simulink model "dynamics"  (R2023b)
settings: Solver=ode45  StartTime=0.0  StopTime=StopTime  FixedStep=.1  RelTol=1e-5
PreLoadFcn:
  | StopTime = 5000; gravity = true; k = 10; b = 100; ktr = 300; btr = 300; d0 = 125; l0 = 515.3882; mu = 398600000000000; mp = 1500; mp_inv = 0.00066667; mtr = 1.6667; mtr_inv = 0.6; NRao0 = [-504.021290494982;4.21156034226775e-10;6878000]; NRbo0 = [504.021290495824;4.21156034226775e-10;6878000]; NRdo0 = [4.21156034226775e-10;-124.968757810126;6878000]; NReo0 = [4.21156034226775e-10;124.968757810969;6878000]; NVao0 = [-7612.67977015526;-3.08624030053628e-16;-5.04021290495356]; NVbo0 = [-7612.67977015526;3.08624030053685e-16;5.04021290495449]; NVdo0 = [-7612.67977015526;2.85429773939059e-29;4.66142195672722e-13]; NVeo0 = [-7612.67977015526;2.85429773939059e-29;4.66142195672722e-13];
undefined symbols (not defined in the file or in its folder): NRfo0, NRgo0, NVfo0, NVgo0
settings Model: Creator=cyrus  LastModifiedBy=cyrus

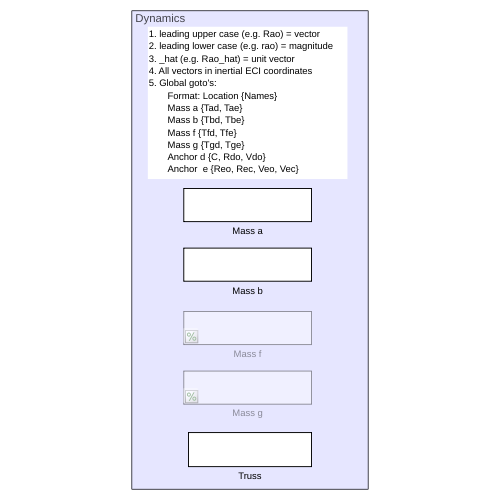
[thumbnail: Simulink's stored preview of the top-level diagram]
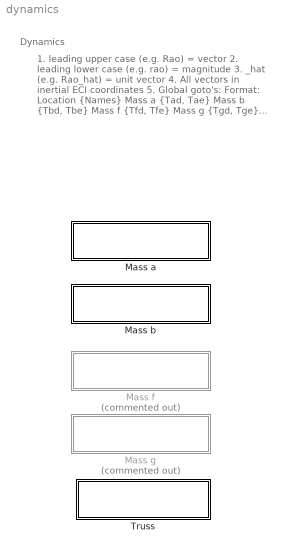
== system dynamics ==
  note: Dynamics
  note: 1. leading upper case (e.g. Rao) = vector
      | 2. leading lower case (e.g. rao) = magnitude
      | 3. _hat (e.g. Rao_hat) = unit vector
      | 4. All vectors in inertial ECI coordinates
      | 5. Global goto's:
      | 	Format: Location {Names}
      | 	Mass a {Tad, Tae}
      | 	Mass b {Tbd, Tbe}
      | 	Mass f {Tfd, Tfe}
      | 	Mass g {Tgd, Tge}
      | 	Anchor d {C, Rdo, Vdo}
      | 	Anchor  e {Reo, Rec, Veo, Vec}
  Mass a : Subsystem
  Mass b : Subsystem
  Mass f : Subsystem  Commented=on
  Mass g : Subsystem  Commented=on
  Truss : Subsystem

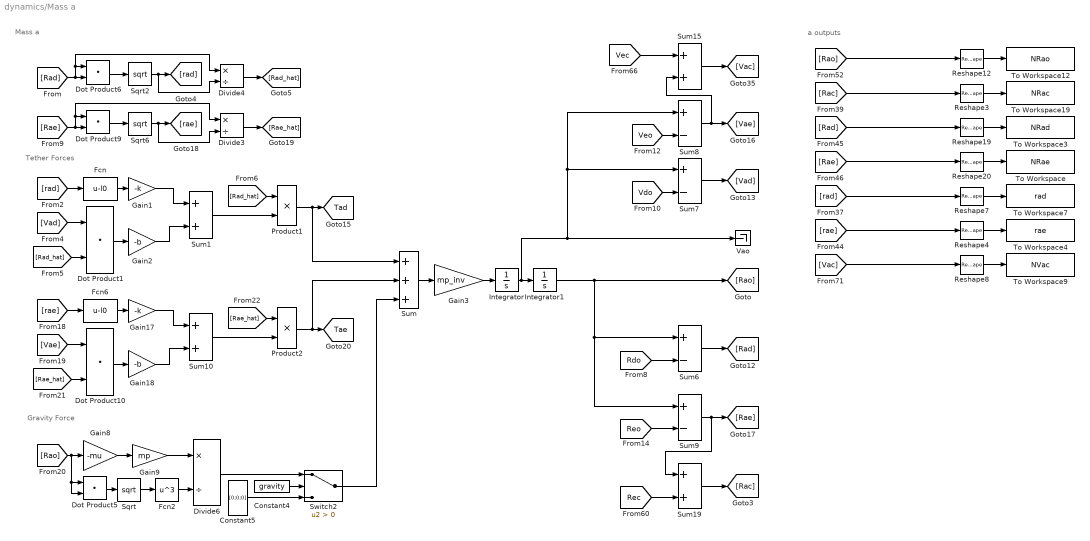
== system dynamics/Mass a ==
  note: Tether Forces
  note: Mass a
  note: Gravity Force
  note: a outputs
  Constant4 : Constant  Value=gravity
  Constant5 : Constant  Value=[0;0;0]  VectorParams1D=off
  Divide3 : Product  Inputs=*/
  Divide4 : Product  Inputs=*/
  Divide6 : Product  Inputs=*/
  Dot Product{1,5..6,9..10} (5 alike) : DotProduct  OutDataTypeStr=Inherit: Inherit via internal rule
  Fcn : Fcn  Expr=u-l0
  Fcn2 : Fcn  Expr=u^3
  Fcn6 : Fcn  Expr=u-l0
  Gain1 : Gain  Gain=-k
  Gain17 : Gain  Gain=-k
  Gain18 : Gain  Gain=-b
  Gain2 : Gain  Gain=-b
  Gain3 : Gain  Gain=mp_inv
  Gain8 : Gain  Gain=-mu
  Gain9 : Gain  Gain=mp
  Integrator : Integrator  InitialCondition=NVao0
  Integrator1 : Integrator  InitialCondition=NRao0
  Product1 : Product
  Product2 : Product
  Reshape{3..4,7..8,12,19..20} (7 alike) : Reshape
  Sqrt : Sqrt
  Sqrt2 : Sqrt
  Sqrt6 : Sqrt
  Sum : Sum  Inputs=+++
  Sum{1,10,15,19} (4 alike) : Sum
  Sum{6..9} (4 alike) : Sum  Inputs=+-
  Switch2 : Switch  Criteria=u2 > Threshold  SaturateOnIntegerOverflow=off  InputSameDT=off
  To Workspace : ToWorkspace  VariableName=NRae  SampleTime=-1
  To Workspace12 : ToWorkspace  VariableName=NRao  SampleTime=-1
      settings: Save2DSignal=2-D array (concatenate along first dimension)
  To Workspace19 : ToWorkspace  VariableName=NRac  SampleTime=-1
      settings: Save2DSignal=2-D array (concatenate along first dimension)
  To Workspace3 : ToWorkspace  VariableName=NRad  SampleTime=-1
  To Workspace4 : ToWorkspace  VariableName=rae  SampleTime=-1
      settings: Save2DSignal=2-D array (concatenate along first dimension)
  To Workspace7 : ToWorkspace  VariableName=rad  SampleTime=-1
      settings: Save2DSignal=2-D array (concatenate along first dimension)
  To Workspace9 : ToWorkspace  VariableName=NVac  SampleTime=-1
      settings: Save2DSignal=2-D array (concatenate along first dimension)
  Vao : Terminator
  tag scope: Tad=global, Tae=global
  wires:
  Sum19/1 -> [Rac]
  [rae] -> Fcn6/1
  [Rdo] -> Sum6/2
  Dot Product6/1 -> Sqrt2/1
  Gain17/1 -> Sum10/1
  [Veo] -> Sum8/2
  [Vec] -> Sum15/1
  Dot Product10/1 -> Gain18/1
  Dot Product5/1 -> Sqrt/1
  Gain18/1 -> Sum10/2
  Sum1/1 -> Product1/2
  Sqrt/1 -> Fcn2/1
  [Rad_hat] -> Product1/1
  Sum9/1 -> Sum19/1, [Rae]
  Constant5/1 -> Switch2/3
  Gain2/1 -> Sum1/2
  Sqrt2/1 -> Divide4/2, [rad]
  Sum8/1 -> Sum15/2, [Vae]
  [Rae_hat] -> Dot Product10/2
  Sum/1 -> Gain3/1
  Integrator1/1 -> [Rao], Sum6/1, Sum9/1
  Fcn2/1 -> Divide6/2
  [rad] -> Fcn/1
  [Rae_hat] -> Product2/1
  Gain3/1 -> Integrator/1
  Gain9/1 -> Divide6/1
  [Rad_hat] -> Dot Product1/2
  Divide4/1 -> [Rad_hat]
  [Rao] -> Dot Product5/2, Dot Product5/1, Gain8/1
  Product2/1 -> Sum/2, [Tae]
  [Rad] -> Divide4/1, Dot Product6/1, Dot Product6/2
  Fcn/1 -> Gain1/1
  Constant4/1 -> Switch2/2
  Gain1/1 -> Sum1/1
  [Vad] -> Dot Product1/1
  Sum10/1 -> Product2/2
  [Reo] -> Sum9/2
  Sum15/1 -> [Vac]
  Dot Product1/1 -> Gain2/1
  Switch2/1 -> Sum/3
  Gain8/1 -> Gain9/1
  Sum7/1 -> [Vad]
  [Rae] -> Divide3/1, Dot Product9/1, Dot Product9/2
  [Rec] -> Sum19/2
  Sqrt6/1 -> Divide3/2, [rae]
  Divide6/1 -> Switch2/1
  [Vdo] -> Sum7/2
  Fcn6/1 -> Gain17/1
  Product1/1 -> Sum/1, [Tad]
  Dot Product9/1 -> Sqrt6/1
  Integrator/1 -> Integrator1/1, Vao/1, Sum7/1, Sum8/1
  Divide3/1 -> [Rae_hat]
  Sum6/1 -> [Rad]
  [Vae] -> Dot Product10/1
  Reshape4/1 -> To Workspace4/1
  Reshape19/1 -> To Workspace3/1
  Reshape8/1 -> To Workspace9/1
  Reshape12/1 -> To Workspace12/1
  [Rad] -> Reshape19/1
  Reshape20/1 -> To Workspace/1
  [Rae] -> Reshape20/1
  [rad] -> Reshape7/1
  Reshape7/1 -> To Workspace7/1
  [Vac] -> Reshape8/1
  [Rao] -> Reshape12/1
  [rae] -> Reshape4/1
  [Rac] -> Reshape3/1
  Reshape3/1 -> To Workspace19/1

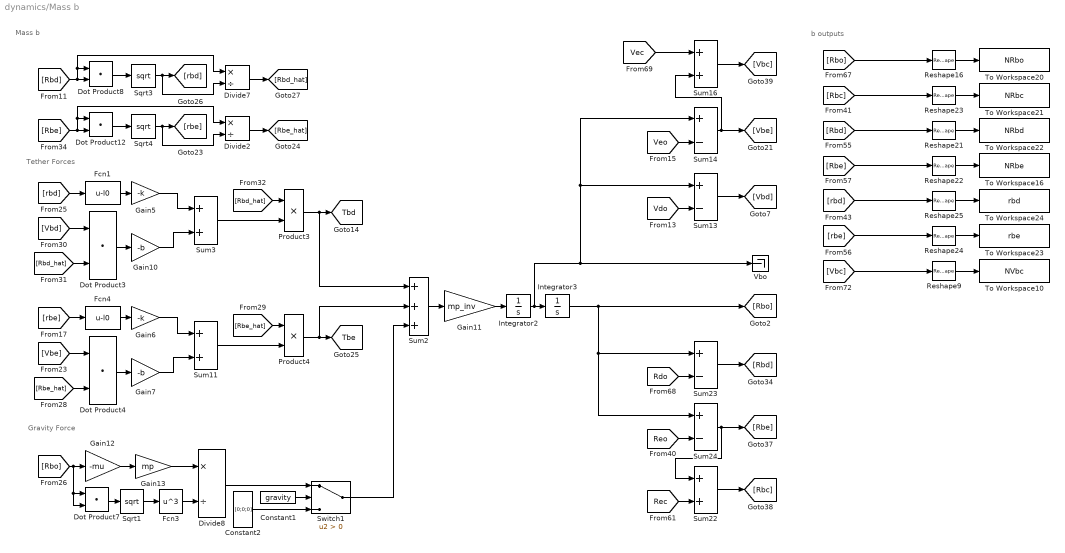
== system dynamics/Mass b ==
  note: Gravity Force
  note: Tether Forces
  note: Mass b
  note: b outputs
  Constant1 : Constant  Value=gravity
  Constant2 : Constant  Value=[0;0;0]  VectorParams1D=off
  Divide2 : Product  Inputs=*/
  Divide7 : Product  Inputs=*/
  Divide8 : Product  Inputs=*/
  Dot Product{3..4,7..8,12} (5 alike) : DotProduct  OutDataTypeStr=Inherit: Inherit via internal rule
  Fcn1 : Fcn  Expr=u-l0
  Fcn3 : Fcn  Expr=u^3
  Fcn4 : Fcn  Expr=u-l0
  Gain10 : Gain  Gain=-b
  Gain11 : Gain  Gain=mp_inv
  Gain12 : Gain  Gain=-mu
  Gain13 : Gain  Gain=mp
  Gain5 : Gain  Gain=-k
  Gain6 : Gain  Gain=-k
  Gain7 : Gain  Gain=-b
  Integrator2 : Integrator  InitialCondition=NVbo0
  Integrator3 : Integrator  InitialCondition=NRbo0
  Product3 : Product
  Product4 : Product
  Reshape{9,16,21..25} (7 alike) : Reshape
  Sqrt1 : Sqrt
  Sqrt3 : Sqrt
  Sqrt4 : Sqrt
  Sum{3,11,16,22} (4 alike) : Sum
  Sum{13..14,23..24} (4 alike) : Sum  Inputs=+-
  Sum2 : Sum  Inputs=+++
  Switch1 : Switch  Criteria=u2 > Threshold  SaturateOnIntegerOverflow=off  InputSameDT=off
  To Workspace10 : ToWorkspace  VariableName=NVbc  SampleTime=-1
      settings: Save2DSignal=2-D array (concatenate along first dimension)
  To Workspace16 : ToWorkspace  VariableName=NRbe  SampleTime=-1
  To Workspace20 : ToWorkspace  VariableName=NRbo  SampleTime=-1
      settings: Save2DSignal=2-D array (concatenate along first dimension)
  To Workspace21 : ToWorkspace  VariableName=NRbc  SampleTime=-1
      settings: Save2DSignal=2-D array (concatenate along first dimension)
  To Workspace22 : ToWorkspace  VariableName=NRbd  SampleTime=-1
  To Workspace23 : ToWorkspace  VariableName=rbe  SampleTime=-1
      settings: Save2DSignal=2-D array (concatenate along first dimension)
  To Workspace24 : ToWorkspace  VariableName=rbd  SampleTime=-1
      settings: Save2DSignal=2-D array (concatenate along first dimension)
  Vbo : Terminator
  tag scope: Tbd=global, Tbe=global
  wires:
  Fcn3/1 -> Divide8/2
  Fcn4/1 -> Gain6/1
  Dot Product12/1 -> Sqrt4/1
  [Rbe_hat] -> Dot Product4/2
  Divide8/1 -> Switch1/1
  Gain12/1 -> Gain13/1
  Sum16/1 -> [Vbc]
  [Vec] -> Sum16/1
  Gain10/1 -> Sum3/2
  Gain13/1 -> Divide8/1
  Product4/1 -> Sum2/2, [Tbe]
  Sum3/1 -> Product3/2
  Dot Product4/1 -> Gain7/1
  Gain11/1 -> Integrator2/1
  [Rbo] -> Dot Product7/2, Dot Product7/1, Gain12/1
  Sum24/1 -> Sum22/1, [Rbe]
  [Rbd] -> Divide7/1, Dot Product8/1, Dot Product8/2
  Sqrt1/1 -> Fcn3/1
  Divide2/1 -> [Rbe_hat]
  Sqrt4/1 -> Divide2/2, [rbe]
  [Rbe_hat] -> Product4/1
  Sum13/1 -> [Vbd]
  Dot Product3/1 -> Gain10/1
  Constant2/1 -> Switch1/3
  [Vdo] -> Sum13/2
  [Rbd_hat] -> Product3/1
  Integrator2/1 -> Integrator3/1, Vbo/1, Sum13/1, Sum14/1
  Constant1/1 -> Switch1/2
  Gain5/1 -> Sum3/1
  Integrator3/1 -> Sum23/1, Sum24/1, [Rbo]
  [Vbd] -> Dot Product3/1
  Gain6/1 -> Sum11/1
  [Rec] -> Sum22/2
  [Vbe] -> Dot Product4/1
  Dot Product7/1 -> Sqrt1/1
  [Veo] -> Sum14/2
  [Rbe] -> Divide2/1, Dot Product12/1, Dot Product12/2
  [Rbd_hat] -> Dot Product3/2
  Sum23/1 -> [Rbd]
  Dot Product8/1 -> Sqrt3/1
  Switch1/1 -> Sum2/3
  [Reo] -> Sum24/2
  Divide7/1 -> [Rbd_hat]
  Sum2/1 -> Gain11/1
  Gain7/1 -> Sum11/2
  Sum22/1 -> [Rbc]
  [rbe] -> Fcn4/1
  Sum11/1 -> Product4/2
  Sum14/1 -> Sum16/2, [Vbe]
  Sqrt3/1 -> Divide7/2, [rbd]
  [rbd] -> Fcn1/1
  Product3/1 -> Sum2/1, [Tbd]
  [Rdo] -> Sum23/2
  Fcn1/1 -> Gain5/1
  Reshape21/1 -> To Workspace22/1
  Reshape23/1 -> To Workspace21/1
  Reshape9/1 -> To Workspace10/1
  [Rbc] -> Reshape23/1
  Reshape25/1 -> To Workspace24/1
  [Vbc] -> Reshape9/1
  Reshape22/1 -> To Workspace16/1
  [Rbo] -> Reshape16/1
  Reshape24/1 -> To Workspace23/1
  [Rbd] -> Reshape21/1
  [rbd] -> Reshape25/1
  [Rbe] -> Reshape22/1
  Reshape16/1 -> To Workspace20/1
  [rbe] -> Reshape24/1

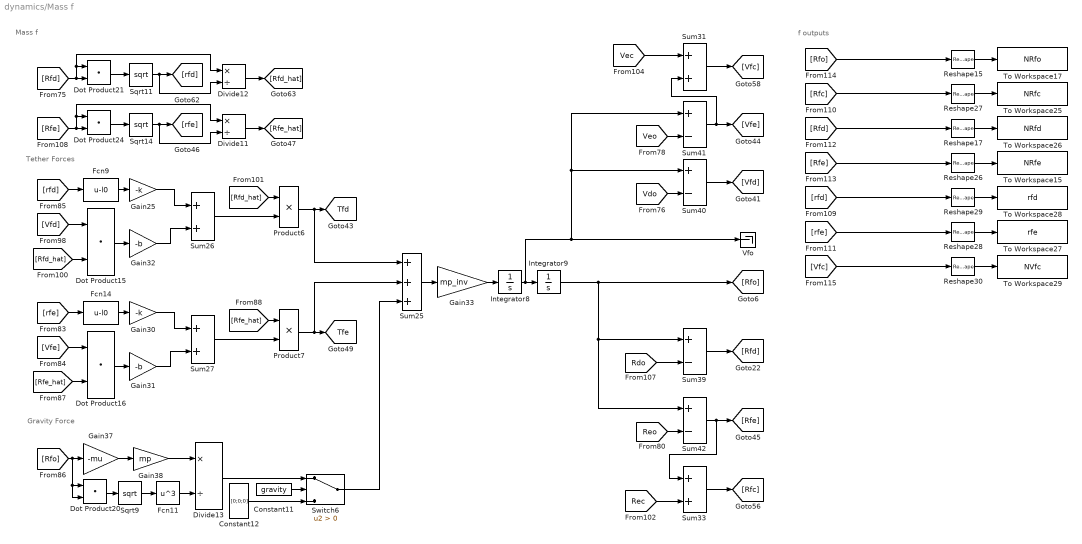
== system dynamics/Mass f ==
  note: Mass f
  note: Tether Forces
  note: Gravity Force
  note: f outputs
  Constant11 : Constant  Value=gravity
  Constant12 : Constant  Value=[0;0;0]  VectorParams1D=off
  Divide11 : Product  Inputs=*/
  Divide12 : Product  Inputs=*/
  Divide13 : Product  Inputs=*/
  Dot Product{15..16,20..21,24} (5 alike) : DotProduct  OutDataTypeStr=Inherit: Inherit via internal rule
  Fcn11 : Fcn  Expr=u^3
  Fcn14 : Fcn  Expr=u-l0
  Fcn9 : Fcn  Expr=u-l0
  Gain25 : Gain  Gain=-k
  Gain30 : Gain  Gain=-k
  Gain31 : Gain  Gain=-b
  Gain32 : Gain  Gain=-b
  Gain33 : Gain  Gain=mp_inv
  Gain37 : Gain  Gain=-mu
  Gain38 : Gain  Gain=mp
  Integrator8 : Integrator  InitialCondition=NVfo0
  Integrator9 : Integrator  InitialCondition=NRfo0
  Product6 : Product
  Product7 : Product
  Reshape{15,17,26..30} (7 alike) : Reshape
  Sqrt11 : Sqrt
  Sqrt14 : Sqrt
  Sqrt9 : Sqrt
  Sum25 : Sum  Inputs=+++
  Sum{26..27,31,33} (4 alike) : Sum
  Sum{39..42} (4 alike) : Sum  Inputs=+-
  Switch6 : Switch  Criteria=u2 > Threshold  SaturateOnIntegerOverflow=off  InputSameDT=off
  To Workspace15 : ToWorkspace  VariableName=NRfe  SampleTime=-1
  To Workspace17 : ToWorkspace  VariableName=NRfo  SampleTime=-1
      settings: Save2DSignal=2-D array (concatenate along first dimension)
  To Workspace25 : ToWorkspace  VariableName=NRfc  SampleTime=-1
      settings: Save2DSignal=2-D array (concatenate along first dimension)
  To Workspace26 : ToWorkspace  VariableName=NRfd  SampleTime=-1
  To Workspace27 : ToWorkspace  VariableName=rfe  SampleTime=-1
      settings: Save2DSignal=2-D array (concatenate along first dimension)
  To Workspace28 : ToWorkspace  VariableName=rfd  SampleTime=-1
      settings: Save2DSignal=2-D array (concatenate along first dimension)
  To Workspace29 : ToWorkspace  VariableName=NVfc  SampleTime=-1
      settings: Save2DSignal=2-D array (concatenate along first dimension)
  Vfo : Terminator
  tag scope: Tfd=global, Tfe=global
  wires:
  [Rec] -> Sum33/2
  Sum27/1 -> Product7/2
  [Vec] -> Sum31/1
  Divide12/1 -> [Rfd_hat]
  Divide13/1 -> Switch6/1
  Sum31/1 -> [Vfc]
  Sum33/1 -> [Rfc]
  [Reo] -> Sum42/2
  Gain33/1 -> Integrator8/1
  Gain25/1 -> Sum26/1
  Sqrt11/1 -> Divide12/2, [rfd]
  Sum41/1 -> Sum31/2, [Vfe]
  Switch6/1 -> Sum25/3
  [rfe] -> Fcn14/1
  Dot Product15/1 -> Gain32/1
  [Vfd] -> Dot Product15/1
  Dot Product21/1 -> Sqrt11/1
  Dot Product20/1 -> Sqrt9/1
  Constant12/1 -> Switch6/3
  [Rfd_hat] -> Dot Product15/2
  Dot Product24/1 -> Sqrt14/1
  [Vdo] -> Sum40/2
  [Veo] -> Sum41/2
  Gain31/1 -> Sum27/2
  [Rfo] -> Dot Product20/2, Dot Product20/1, Gain37/1
  [Rfd_hat] -> Product6/1
  [Rfe] -> Divide11/1, Dot Product24/1, Dot Product24/2
  Fcn14/1 -> Gain30/1
  Integrator9/1 -> [Rfo], Sum39/1, Sum42/1
  Integrator8/1 -> Integrator9/1, Vfo/1, Sum40/1, Sum41/1
  Sqrt9/1 -> Fcn11/1
  Product6/1 -> Sum25/1, [Tfd]
  Gain32/1 -> Sum26/2
  Product7/1 -> Sum25/2, [Tfe]
  [Rfe_hat] -> Dot Product16/2
  Sum40/1 -> [Vfd]
  Sum42/1 -> Sum33/1, [Rfe]
  [Rdo] -> Sum39/2
  [Rfd] -> Divide12/1, Dot Product21/1, Dot Product21/2
  Fcn9/1 -> Gain25/1
  [Rfe_hat] -> Product7/1
  Gain37/1 -> Gain38/1
  Gain38/1 -> Divide13/1
  Sqrt14/1 -> Divide11/2, [rfe]
  Sum26/1 -> Product6/2
  Divide11/1 -> [Rfe_hat]
  Fcn11/1 -> Divide13/2
  Sum25/1 -> Gain33/1
  [Vfe] -> Dot Product16/1
  Sum39/1 -> [Rfd]
  [rfd] -> Fcn9/1
  Gain30/1 -> Sum27/1
  Constant11/1 -> Switch6/2
  Dot Product16/1 -> Gain31/1
  Reshape26/1 -> To Workspace15/1
  [Vfc] -> Reshape30/1
  Reshape30/1 -> To Workspace29/1
  [Rfe] -> Reshape26/1
  Reshape27/1 -> To Workspace25/1
  [Rfd] -> Reshape17/1
  Reshape29/1 -> To Workspace28/1
  [rfe] -> Reshape28/1
  Reshape28/1 -> To Workspace27/1
  [Rfc] -> Reshape27/1
  [Rfo] -> Reshape15/1
  Reshape17/1 -> To Workspace26/1
  [rfd] -> Reshape29/1
  Reshape15/1 -> To Workspace17/1

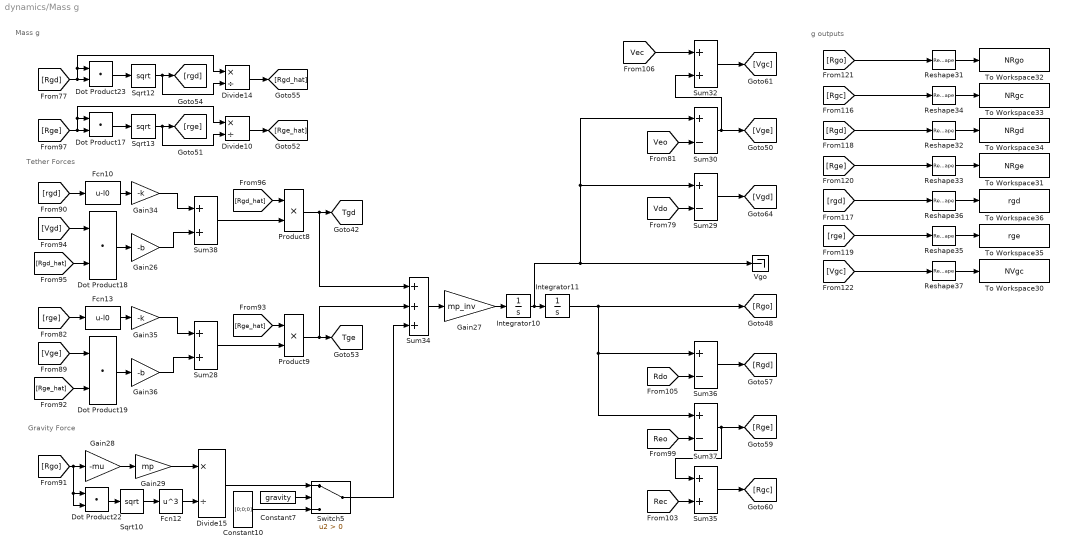
== system dynamics/Mass g ==
  note: Mass g
  note: Tether Forces
  note: Gravity Force
  note: g outputs
  Constant10 : Constant  Value=[0;0;0]  VectorParams1D=off
  Constant7 : Constant  Value=gravity
  Divide10 : Product  Inputs=*/
  Divide14 : Product  Inputs=*/
  Divide15 : Product  Inputs=*/
  Dot Product{17..19,22..23} (5 alike) : DotProduct  OutDataTypeStr=Inherit: Inherit via internal rule
  Fcn10 : Fcn  Expr=u-l0
  Fcn12 : Fcn  Expr=u^3
  Fcn13 : Fcn  Expr=u-l0
  Gain26 : Gain  Gain=-b
  Gain27 : Gain  Gain=mp_inv
  Gain28 : Gain  Gain=-mu
  Gain29 : Gain  Gain=mp
  Gain34 : Gain  Gain=-k
  Gain35 : Gain  Gain=-k
  Gain36 : Gain  Gain=-b
  Integrator10 : Integrator  InitialCondition=NVgo0
  Integrator11 : Integrator  InitialCondition=NRgo0
  Product8 : Product
  Product9 : Product
  Reshape{31..37} (7 alike) : Reshape
  Sqrt10 : Sqrt
  Sqrt12 : Sqrt
  Sqrt13 : Sqrt
  Sum{28,32,35,38} (4 alike) : Sum
  Sum{29..30,36..37} (4 alike) : Sum  Inputs=+-
  Sum34 : Sum  Inputs=+++
  Switch5 : Switch  Criteria=u2 > Threshold  SaturateOnIntegerOverflow=off  InputSameDT=off
  To Workspace30 : ToWorkspace  VariableName=NVgc  SampleTime=-1
      settings: Save2DSignal=2-D array (concatenate along first dimension)
  To Workspace31 : ToWorkspace  VariableName=NRge  SampleTime=-1
  To Workspace32 : ToWorkspace  VariableName=NRgo  SampleTime=-1
      settings: Save2DSignal=2-D array (concatenate along first dimension)
  To Workspace33 : ToWorkspace  VariableName=NRgc  SampleTime=-1
      settings: Save2DSignal=2-D array (concatenate along first dimension)
  To Workspace34 : ToWorkspace  VariableName=NRgd  SampleTime=-1
  To Workspace35 : ToWorkspace  VariableName=rge  SampleTime=-1
      settings: Save2DSignal=2-D array (concatenate along first dimension)
  To Workspace36 : ToWorkspace  VariableName=rgd  SampleTime=-1
      settings: Save2DSignal=2-D array (concatenate along first dimension)
  Vgo : Terminator
  tag scope: Tgd=global, Tge=global
  wires:
  Sum36/1 -> [Rgd]
  Gain29/1 -> Divide15/1
  [Rge_hat] -> Product9/1
  Sum34/1 -> Gain27/1
  Sqrt10/1 -> Fcn12/1
  Dot Product22/1 -> Sqrt10/1
  [rge] -> Fcn13/1
  [Veo] -> Sum30/2
  Switch5/1 -> Sum34/3
  Gain27/1 -> Integrator10/1
  Gain35/1 -> Sum28/1
  Fcn12/1 -> Divide15/2
  [rgd] -> Fcn10/1
  Product8/1 -> Sum34/1, [Tgd]
  [Vgd] -> Dot Product18/1
  Constant10/1 -> Switch5/3
  Gain34/1 -> Sum38/1
  Gain26/1 -> Sum38/2
  Product9/1 -> Sum34/2, [Tge]
  Sqrt13/1 -> Divide10/2, [rge]
  [Rge_hat] -> Dot Product19/2
  [Rgd_hat] -> Product8/1
  [Rgd] -> Divide14/1, Dot Product23/1, Dot Product23/2
  Divide15/1 -> Switch5/1
  Sum37/1 -> Sum35/1, [Rge]
  [Rge] -> Divide10/1, Dot Product17/1, Dot Product17/2
  Integrator10/1 -> Integrator11/1, Vgo/1, Sum29/1, Sum30/1
  Sum38/1 -> Product8/2
  Integrator11/1 -> Sum36/1, Sum37/1, [Rgo]
  Sum28/1 -> Product9/2
  [Rec] -> Sum35/2
  Constant7/1 -> Switch5/2
  Sum29/1 -> [Vgd]
  [Rgo] -> Dot Product22/2, Dot Product22/1, Gain28/1
  Gain28/1 -> Gain29/1
  Gain36/1 -> Sum28/2
  [Rgd_hat] -> Dot Product18/2
  [Vec] -> Sum32/1
  [Rdo] -> Sum36/2
  Divide10/1 -> [Rge_hat]
  Sum30/1 -> Sum32/2, [Vge]
  Fcn10/1 -> Gain34/1
  [Vge] -> Dot Product19/1
  Sum32/1 -> [Vgc]
  [Reo] -> Sum37/2
  Divide14/1 -> [Rgd_hat]
  Dot Product23/1 -> Sqrt12/1
  Dot Product19/1 -> Gain36/1
  [Vdo] -> Sum29/2
  Dot Product18/1 -> Gain26/1
  Sum35/1 -> [Rgc]
  Sqrt12/1 -> Divide14/2, [rgd]
  Fcn13/1 -> Gain35/1
  Dot Product17/1 -> Sqrt13/1
  Reshape33/1 -> To Workspace31/1
  Reshape37/1 -> To Workspace30/1
  Reshape36/1 -> To Workspace36/1
  Reshape31/1 -> To Workspace32/1
  [Rgc] -> Reshape34/1
  [rge] -> Reshape35/1
  [rgd] -> Reshape36/1
  [Rgo] -> Reshape31/1
  [Rgd] -> Reshape32/1
  Reshape32/1 -> To Workspace34/1
  Reshape35/1 -> To Workspace35/1
  Reshape34/1 -> To Workspace33/1
  [Rge] -> Reshape33/1
  [Vgc] -> Reshape37/1

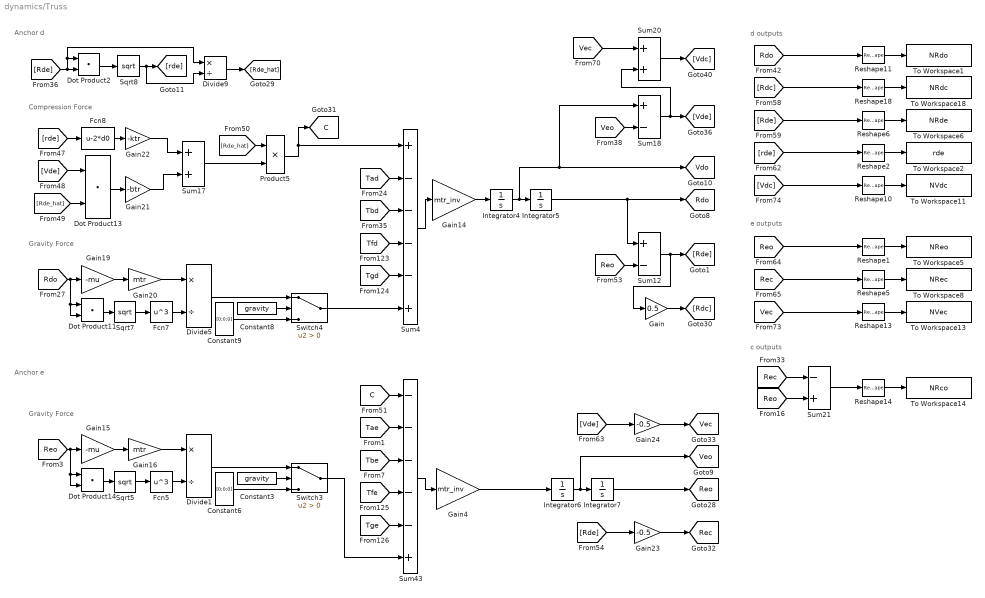
== system dynamics/Truss ==
  note: Anchor d
  note: Gravity Force
  note: Compression Force
  note: d outputs
  note: Gravity Force
  note: Anchor e
  note: e outputs
  note: c outputs
  Constant3 : Constant  Value=gravity
  Constant6 : Constant  Value=[0;0;0]  VectorParams1D=off
  Constant8 : Constant  Value=gravity
  Constant9 : Constant  Value=[0;0;0]  VectorParams1D=off
  Divide1 : Product  Inputs=*/
  Divide5 : Product  Inputs=*/
  Divide9 : Product  Inputs=*/
  Dot Product{2,11,13..14} (4 alike) : DotProduct  OutDataTypeStr=Inherit: Inherit via internal rule
  Fcn5 : Fcn  Expr=u^3
  Fcn7 : Fcn  Expr=u^3
  Fcn8 : Fcn  Expr=u-2*d0
  Gain : Gain  Gain=0.5
  Gain14 : Gain  Gain=mtr_inv
  Gain15 : Gain  Gain=-mu
  Gain16 : Gain  Gain=mtr
  Gain19 : Gain  Gain=-mu
  Gain20 : Gain  Gain=mtr
  Gain21 : Gain  Gain=-btr
  Gain22 : Gain  Gain=-ktr
  Gain23 : Gain  Gain=-0.5
  Gain24 : Gain  Gain=-0.5
  Gain4 : Gain  Gain=mtr_inv
  Integrator4 : Integrator  InitialCondition=NVdo0
  Integrator5 : Integrator  InitialCondition=NRdo0
  Integrator6 : Integrator  InitialCondition=NVeo0
  Integrator7 : Integrator  InitialCondition=NReo0
  Product5 : Product
  Reshape{1..2,5..6,10..11,13..14,18} (9 alike) : Reshape
  Sqrt5 : Sqrt
  Sqrt7 : Sqrt
  Sqrt8 : Sqrt
  Sum12 : Sum  Inputs=+-
  Sum17 : Sum
  Sum18 : Sum  Inputs=+-
  Sum20 : Sum
  Sum21 : Sum  Inputs=-+
  Sum4 : Sum  Inputs=+----+
  Sum43 : Sum  Inputs=-----+
  Switch3 : Switch  Criteria=u2 > Threshold  SaturateOnIntegerOverflow=off  InputSameDT=off
  Switch4 : Switch  Criteria=u2 > Threshold  SaturateOnIntegerOverflow=off  InputSameDT=off
  To Workspace1 : ToWorkspace  VariableName=NRdo  SampleTime=-1
      settings: Save2DSignal=2-D array (concatenate along first dimension)
  To Workspace11 : ToWorkspace  VariableName=NVdc  SampleTime=-1
      settings: Save2DSignal=2-D array (concatenate along first dimension)
  To Workspace13 : ToWorkspace  VariableName=NVec  SampleTime=-1
      settings: Save2DSignal=2-D array (concatenate along first dimension)
  To Workspace14 : ToWorkspace  VariableName=NRco  SampleTime=-1
      settings: Save2DSignal=2-D array (concatenate along first dimension)
  To Workspace18 : ToWorkspace  VariableName=NRdc  SampleTime=-1
      settings: Save2DSignal=2-D array (concatenate along first dimension)
  To Workspace2 : ToWorkspace  VariableName=rde  SampleTime=-1
      settings: Save2DSignal=2-D array (concatenate along first dimension)
  To Workspace5 : ToWorkspace  VariableName=NReo  SampleTime=-1
      settings: Save2DSignal=2-D array (concatenate along first dimension)
  To Workspace6 : ToWorkspace  VariableName=NRde  SampleTime=-1
      settings: Save2DSignal=2-D array (concatenate along first dimension)
  To Workspace8 : ToWorkspace  VariableName=NRec  SampleTime=-1
      settings: Save2DSignal=2-D array (concatenate along first dimension)
  tag scope: C=global, Rdo=global, Rec=global, Reo=global, Vdo=global, Vec=global, Veo=global
  wires:
  [Veo] -> Sum18/2
  [Tad] -> Sum4/2
  [Tbd] -> Sum4/3
  Constant8/1 -> Switch4/2
  Sum4/1 -> Gain14/1
  Gain14/1 -> Integrator4/1
  Constant9/1 -> Switch4/3
  Product5/1 -> [C], Sum4/1
  Gain/1 -> [Rdc]
  [Tgd] -> Sum4/5
  Fcn8/1 -> Gain22/1
  Integrator5/1 -> Sum12/1, [Rdo]
  [Vde] -> Dot Product13/1
  Gain22/1 -> Sum17/1
  Fcn7/1 -> Divide5/2
  [Rde_hat] -> Dot Product13/2
  [Rde_hat] -> Product5/1
  Gain20/1 -> Divide5/1
  [Reo] -> Sum12/2
  Sum12/1 -> Gain/1, [Rde]
  Integrator4/1 -> Sum18/1, [Vdo], Integrator5/1
  Divide5/1 -> Switch4/1
  [Vec] -> Sum20/1
  [Tfd] -> Sum4/4
  Sqrt8/1 -> Divide9/2, [rde]
  Sqrt7/1 -> Fcn7/1
  [Rde] -> Divide9/1, Dot Product2/1, Dot Product2/2
  Sum18/1 -> Sum20/2, [Vde]
  Sum20/1 -> [Vdc]
  Switch4/1 -> Sum4/6
  [Rdo] -> Dot Product11/2, Dot Product11/1, Gain19/1
  Dot Product11/1 -> Sqrt7/1
  Gain19/1 -> Gain20/1
  Sum17/1 -> Product5/2
  Dot Product2/1 -> Sqrt8/1
  Dot Product13/1 -> Gain21/1
  Divide9/1 -> [Rde_hat]
  Gain21/1 -> Sum17/2
  [rde] -> Fcn8/1
  [Vdc] -> Reshape10/1
  [Rdo] -> Reshape11/1
  [rde] -> Reshape2/1
  [Rde] -> Reshape6/1
  Reshape10/1 -> To Workspace11/1
  Reshape6/1 -> To Workspace6/1
  Reshape18/1 -> To Workspace18/1
  Reshape11/1 -> To Workspace1/1
  [Rdc] -> Reshape18/1
  Reshape2/1 -> To Workspace2/1
  Sqrt5/1 -> Fcn5/1
  Dot Product14/1 -> Sqrt5/1
  Divide1/1 -> Switch3/1
  Gain4/1 -> Integrator6/1
  Integrator7/1 -> [Reo]
  [Rde] -> Gain23/1
  Sum43/1 -> Gain4/1
  [Tae] -> Sum43/2
  Gain16/1 -> Divide1/1
  [Tbe] -> Sum43/3
  Reshape13/1 -> To Workspace13/1
  Fcn5/1 -> Divide1/2
  [Tge] -> Sum43/5
  [Vde] -> Gain24/1
  Switch3/1 -> Sum43/6
  Gain15/1 -> Gain16/1
  [Tfe] -> Sum43/4
  Constant3/1 -> Switch3/2
  Reshape1/1 -> To Workspace5/1
  Integrator6/1 -> [Veo], Integrator7/1
  Reshape5/1 -> To Workspace8/1
  Gain24/1 -> [Vec]
  [Reo] -> Reshape1/1
  [Vec] -> Reshape13/1
  Constant6/1 -> Switch3/3
  Gain23/1 -> [Rec]
  [Rec] -> Reshape5/1
  [C] -> Sum43/1
  [Reo] -> Dot Product14/2, Dot Product14/1, Gain15/1
  [Rec] -> Sum21/1
  [Reo] -> Sum21/2
  Sum21/1 -> Reshape14/1
  Reshape14/1 -> To Workspace14/1
